simulink model "nms_model_Push"  (R2019a)
settings: Solver=ode15s  StartTime=0.0  StopTime=10  FixedStep=1e-3  MaxStep=ts_max  RelTol=1e-3  AbsTol=1e-4  EnableMultiTasking=on
InitFcn:
  | nms_model_MechInit
  | nms_model_ControlInit
values from neighbouring files (symbols this model uses):
  GainDeltaTheta = 2 /100*180/pi    (= 1.14591559026)    [nms_model_ControlInit.m]
  GainGAS = 1.1/FmaxGAS    [nms_model_ControlInit.m]
  GainGLU = 0.5/FmaxGLU    [nms_model_ControlInit.m]
  GainHAM = 0.65/FmaxHAM    [nms_model_ControlInit.m]
  GainHAMHFL = 4    [nms_model_ControlInit.m]
  GainHFL = 0.5    [nms_model_ControlInit.m]
  GainKneOverExt = 2    [nms_model_ControlInit.m]
  GainSOL = 1.2/FmaxSOL    [nms_model_ControlInit.m]
  GainSOLTA = 0.4/FmaxSOL    [nms_model_ControlInit.m]
  GainTA = 1.1    [nms_model_ControlInit.m]
  GainVAS = 1.2/FmaxVAS    [nms_model_ControlInit.m]
  K_swing = 0.25    [nms_model_ControlInit.m]
  KneePh23Offset = 170*pi/180    (= 2.96705972839)    [nms_model_ControlInit.m]
  LceOffsetHAM = 0.85    [nms_model_ControlInit.m]
  LceOffsetHFL = 0.65    [nms_model_ControlInit.m]
  LceOffsetTA = 1-0.5*w    [nms_model_ControlInit.m]
  LongDelay = 0.020    (= 0.02)    [nms_model_ControlInit.m]
  MidDelay = 0.010    (= 0.01)    [nms_model_ControlInit.m]
  PosGainGG = 1/(30*pi/180)    (= 1.9098593171)    [nms_model_ControlInit.m]
  PreStimGAS = 0.01    [nms_model_ControlInit.m]
  PreStimGG = 0.05    [nms_model_ControlInit.m]
  PreStimGLU = 0.01    [nms_model_ControlInit.m]
  PreStimHAM = 0.01    [nms_model_ControlInit.m]
  PreStimHFL = 0.01    [nms_model_ControlInit.m]
  PreStimSOL = 0.01    [nms_model_ControlInit.m]
  PreStimTA = 0.01    [nms_model_ControlInit.m]
  PreStimVAS = 0.08    [nms_model_ControlInit.m]
  ShortDelay = 0.005    [nms_model_ControlInit.m]
  SpeedGainGG = 0.2    [nms_model_ControlInit.m]
  Theta0 = 6*pi/180    (= 0.10471975512)    [nms_model_ControlInit.m]
undefined symbols (not defined in the file or in its folder): c, c_jointstop, D12_F, D12_S, D12_T, D13_F, D1G_F, D1G_HAT, D1G_S, D1G_T, DeltaThRef, disturbances, dt_visual, eref, FmaxGAS, FmaxGLU, FmaxHAM, FmaxHFL, FmaxSOL, FmaxTA, FmaxVAS, In_F, In_HAT, In_S, In_T, K, k_gx, k_gy, k_pressure, loptGAS, loptGLU, loptHAM, loptHFL, loptSOL, loptTA, loptVAS, lslackGAS, lslackGLU, lslackHAM, lslackHFL, lslackSOL, lslackTA, lslackVAS, m_F, m_HAT, m_S, m_T, mu_slide, mu_stick, N, phi12_LowLimit, phi12_UpLimit, phi23_UpLimit, phi34_UpLimit, phimaxGASa, phimaxGASk, phimaxHAMk, phimaxSOL, phimaxTA, phimaxVAS ... (+44)
libraries: mblibv1 x69, simulink x22, simulink_extras x20, myLibrary2019a x3, myLibrary x1
(part 4 of 8)

== system nms_model_Push/Muscle Actuation Layer/L GAS ==
  note: SOLEUS Muscle-Tendon Dynamics
  note: Excitation Contraction Coupling
  STIM : Inport
  lmtc [m] : Inport  Port=2
  1 : Product  Inputs=**  SaturateOnIntegerOverflow=on  InputSameDT=on  OutDataTypeStr=Inherit: Same as first input
  1/lslack : Gain  Gain=1/lslackGAS  SaturateOnIntegerOverflow=on  OutDataTypeStr=Inherit: Same as input  ParamDataTypeStr=Inherit: Same as input
  BE force-length relation : Subsystem
  CE force-length relation : Subsystem
  CE inverse force-velocity relation : Subsystem
  Constant : Constant  Value=lslackGAS
  ECC TransferFcn : simulink_extras/Additional Linear/Transfer Fcn (with initial outputs)  N=[1]  D="[tau  1]"  Y0=preA  U0=0
      settings: AttributesFormatString=pre-activation: %<Y0>
  Fmax : Gain  Gain=FmaxGAS  SaturateOnIntegerOverflow=on  OutDataTypeStr=Inherit: Same as input  ParamDataTypeStr=Inherit: Same as input
  Fv = Fse / (A*Fce) : Product  Inputs=*/  SaturateOnIntegerOverflow=on  InputSameDT=on  OutDataTypeStr=Inherit: Same as first input
  Integrator : Integrator  InitialConditionSource=external  LowerSaturationLimit=0.05
  PE force-length relation : Subsystem
  SE force-length relation : Subsystem
  Sum : Sum  Inputs=|+-  SaturateOnIntegerOverflow=on  InputSameDT=on  OutDataTypeStr=Inherit: Same as first input
  Sum2 : Sum  Inputs=|-+  SaturateOnIntegerOverflow=on  InputSameDT=on  OutDataTypeStr=Inherit: Same as first input
  Sum3 : Sum  SaturateOnIntegerOverflow=on  InputSameDT=on  OutDataTypeStr=Inherit: Same as first input
  Sum4 : Sum  SaturateOnIntegerOverflow=on  InputSameDT=on  OutDataTypeStr=Inherit: Same as first input
  lce/lopt : Gain  Gain=1/loptGAS  SaturateOnIntegerOverflow=on  OutDataTypeStr=Inherit: Same as input  ParamDataTypeStr=Inherit: Same as input
  vmax*lopt : Gain  Gain=vmaxGAS*loptGAS  SaturateOnIntegerOverflow=on  OutDataTypeStr=Inherit: Same as input  ParamDataTypeStr=Inherit: Same as input
  Fmtc : Outport  InitialOutput=0  VectorParamsAs1DForOutWhenUnconnected=on
  Lce : Outport  Port=2  InitialOutput=0  VectorParamsAs1DForOutWhenUnconnected=on
  Vce : Outport  Port=3  InitialOutput=0  VectorParamsAs1DForOutWhenUnconnected=on
  Lse : Outport  Port=4  InitialOutput=0  VectorParamsAs1DForOutWhenUnconnected=on
  A : Outport  Port=5  InitialOutput=0  VectorParamsAs1DForOutWhenUnconnected=on
  wires:
  Integrator/1 -> Sum/2, lce/lopt/1, Lce/1  "lce"
  Sum/1 -> 1/lslack/1, Lse/1  "lse"
  lce/lopt/1 -> CE force-length relation/1(lce [lopt]), BE force-length relation/1(lce [lopt]), PE force-length relation/1(lce [lopt])
  Fv = Fse / (A*Fce)/1 -> CE inverse force-velocity relation/1(Fv[Fmax])  "fv"
  vmax*lopt/1 -> Integrator/1, Vce/1  "vce"
  lmtc [m]/1 -> Sum2/2, Sum/1  "lmtc"
  Fmax/1 -> Fmtc/1  "Fmtc"
  1/lslack/1 -> SE force-length relation/1(lse [lslack])
  SE force-length relation/1(fse [Fmax]) -> Fmax/1, Sum4/1
  Sum2/1 -> Integrator/2
  Constant/1 -> Sum2/1
  CE force-length relation/1(fce [Fmax]) -> 1/1
  Sum4/1 -> Fv = Fse / (A*Fce)/1
  PE force-length relation/1(fpe [Fmax]) -> Sum3/1
  1/1 -> Sum3/2
  BE force-length relation/1(fbe [Fmax]) -> Sum4/2
  Sum3/1 -> Fv = Fse / (A*Fce)/2
  CE inverse force-velocity relation/1(v[vmax]) -> vmax*lopt/1
  STIM/1 -> ECC TransferFcn/1
  ECC TransferFcn/1 -> A/1, 1/2

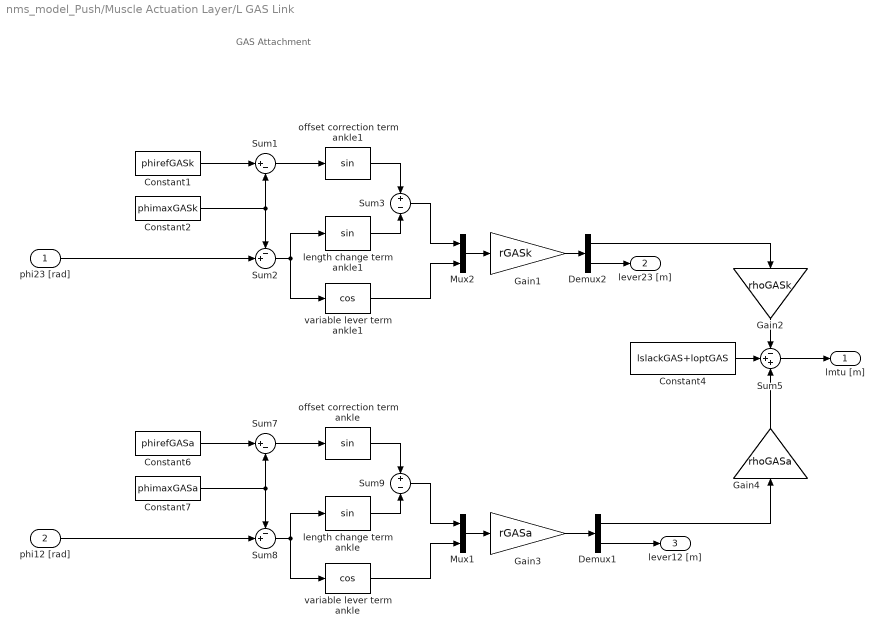
== system nms_model_Push/Muscle Actuation Layer/L GAS Link ==
  note: GAS Attachment
  phi23 [rad] : Inport
  phi12 [rad] : Inport  Port=2
  Constant1 : Constant  Value=phirefGASk
  Constant2 : Constant  Value=phimaxGASk
  Constant4 : Constant  Value=lslackGAS+loptGAS
  Constant6 : Constant  Value=phirefGASa
  Constant7 : Constant  Value=phimaxGASa
  Demux1 : Demux  Outputs=2
  Demux2 : Demux  Outputs=2
  Gain1 : Gain  Gain=rGASk
  Gain2 : Gain  Gain=rhoGASk
  Gain3 : Gain  Gain=rGASa
  Gain4 : Gain  Gain=rhoGASa
  Mux1 : Mux  Inputs=2
  Mux2 : Mux  Inputs=2
  Sum1 : Sum  Inputs=|+-
  Sum2 : Sum  Inputs=-+|
  Sum3 : Sum  Inputs=+-
  Sum5 : Sum  Inputs=-++
  Sum7 : Sum  Inputs=|+-
  Sum8 : Sum  Inputs=-+|
  Sum9 : Sum  Inputs=+-
  length change term ankle : Trigonometry
  length change term ankle1 : Trigonometry
  offset correction term ankle : Trigonometry
  offset correction term ankle1 : Trigonometry
  variable lever term ankle : Trigonometry  Operator=cos
  variable lever term ankle1 : Trigonometry  Operator=cos
  lmtu [m] : Outport  VectorParamsAs1DForOutWhenUnconnected=on
  lever23 [m] : Outport  Port=2  VectorParamsAs1DForOutWhenUnconnected=on
  lever12 [m] : Outport  Port=3  VectorParamsAs1DForOutWhenUnconnected=on
  wires:
  phi12 [rad]/1 -> Sum8/2
  Sum5/1 -> lmtu [m]/1
  variable lever term ankle/1 -> Mux1/2
  Demux1/2 -> lever12 [m]/1
  Sum8/1 -> variable lever term ankle/1, length change term ankle/1
  Constant7/1 -> Sum8/1, Sum7/2
  Sum7/1 -> offset correction term ankle/1
  Constant6/1 -> Sum7/1
  length change term ankle/1 -> Sum9/2
  offset correction term ankle/1 -> Sum9/1
  Sum9/1 -> Mux1/1
  Constant4/1 -> Sum5/2
  Mux1/1 -> Gain3/1
  Gain3/1 -> Demux1/1
  Demux1/1 -> Gain4/1
  Gain4/1 -> Sum5/3
  phi23 [rad]/1 -> Sum2/2
  variable lever term ankle1/1 -> Mux2/2
  Sum2/1 -> variable lever term ankle1/1, length change term ankle1/1
  Constant2/1 -> Sum2/1, Sum1/2
  Sum1/1 -> offset correction term ankle1/1
  Constant1/1 -> Sum1/1
  length change term ankle1/1 -> Sum3/2
  offset correction term ankle1/1 -> Sum3/1
  Sum3/1 -> Mux2/1
  Mux2/1 -> Gain1/1
  Gain1/1 -> Demux2/1
  Demux2/2 -> lever23 [m]/1
  Demux2/1 -> Gain2/1
  Gain2/1 -> Sum5/1

== system nms_model_Push/Muscle Actuation Layer/L GLU ==
  note: SOLEUS Muscle-Tendon Dynamics
  note: Excitation Contraction Coupling
  STIM : Inport
  lmtc [m] : Inport  Port=2
  1 : Product  Inputs=**  SaturateOnIntegerOverflow=on  InputSameDT=on  OutDataTypeStr=Inherit: Same as first input
  1/lslack : Gain  Gain=1/lslackGLU  SaturateOnIntegerOverflow=on  OutDataTypeStr=Inherit: Same as input  ParamDataTypeStr=Inherit: Same as input
  BE force-length relation : Subsystem
  CE force-length relation : Subsystem
  CE inverse force-velocity relation : Subsystem
  Constant : Constant  Value=lslackGLU
  ECC TransferFcn : simulink_extras/Additional Linear/Transfer Fcn (with initial outputs)  N=[1]  D="[tau  1]"  Y0=preA  U0=0
      settings: AttributesFormatString=pre-activation: %<Y0>
  Fmax : Gain  Gain=FmaxGLU  SaturateOnIntegerOverflow=on  OutDataTypeStr=Inherit: Same as input  ParamDataTypeStr=Inherit: Same as input
  Fv = Fse / (A*Fce) : Product  Inputs=*/  SaturateOnIntegerOverflow=on  InputSameDT=on  OutDataTypeStr=Inherit: Same as first input
  Integrator : Integrator  InitialConditionSource=external  LowerSaturationLimit=0.05
  PE force-length relation : Subsystem
  SE force-length relation : Subsystem
  Sum : Sum  Inputs=|+-  SaturateOnIntegerOverflow=on  InputSameDT=on  OutDataTypeStr=Inherit: Same as first input
  Sum2 : Sum  Inputs=|-+  SaturateOnIntegerOverflow=on  InputSameDT=on  OutDataTypeStr=Inherit: Same as first input
  Sum3 : Sum  SaturateOnIntegerOverflow=on  InputSameDT=on  OutDataTypeStr=Inherit: Same as first input
  Sum4 : Sum  SaturateOnIntegerOverflow=on  InputSameDT=on  OutDataTypeStr=Inherit: Same as first input
  lce/lopt : Gain  Gain=1/loptGLU  SaturateOnIntegerOverflow=on  OutDataTypeStr=Inherit: Same as input  ParamDataTypeStr=Inherit: Same as input
  vmax*lopt : Gain  Gain=vmaxGLU*loptGLU  SaturateOnIntegerOverflow=on  OutDataTypeStr=Inherit: Same as input  ParamDataTypeStr=Inherit: Same as input
  Fmtc : Outport  InitialOutput=0  VectorParamsAs1DForOutWhenUnconnected=on
  Lce : Outport  Port=2  InitialOutput=0  VectorParamsAs1DForOutWhenUnconnected=on
  Vce : Outport  Port=3  InitialOutput=0  VectorParamsAs1DForOutWhenUnconnected=on
  Lse : Outport  Port=4  InitialOutput=0  VectorParamsAs1DForOutWhenUnconnected=on
  A : Outport  Port=5  InitialOutput=0  VectorParamsAs1DForOutWhenUnconnected=on
  wires:
  Integrator/1 -> Sum/2, lce/lopt/1, Lce/1  "lce"
  Sum/1 -> 1/lslack/1, Lse/1  "lse"
  lce/lopt/1 -> CE force-length relation/1(lce [lopt]), BE force-length relation/1(lce [lopt]), PE force-length relation/1(lce [lopt])
  Fv = Fse / (A*Fce)/1 -> CE inverse force-velocity relation/1(Fv[Fmax])  "fv"
  vmax*lopt/1 -> Integrator/1, Vce/1  "vce"
  lmtc [m]/1 -> Sum2/2, Sum/1  "lmtc"
  Fmax/1 -> Fmtc/1  "Fmtc"
  1/lslack/1 -> SE force-length relation/1(lse [lslack])
  SE force-length relation/1(fse [Fmax]) -> Fmax/1, Sum4/1
  Sum2/1 -> Integrator/2
  Constant/1 -> Sum2/1
  CE force-length relation/1(fce [Fmax]) -> 1/1
  Sum4/1 -> Fv = Fse / (A*Fce)/1
  PE force-length relation/1(fpe [Fmax]) -> Sum3/1
  1/1 -> Sum3/2
  BE force-length relation/1(fbe [Fmax]) -> Sum4/2
  Sum3/1 -> Fv = Fse / (A*Fce)/2
  CE inverse force-velocity relation/1(v[vmax]) -> vmax*lopt/1
  STIM/1 -> ECC TransferFcn/1
  ECC TransferFcn/1 -> A/1, 1/2

== system nms_model_Push/Muscle Actuation Layer/L GLU Link ==
  note: GLUTEUS Attachment
  phi34 [rad] : Inport
  Constant : Constant  Value=lslackGLU+loptGLU
  Constant1 : Constant  Value=rGLU
  Constant2 : Constant  Value=phirefGLU
  Gain2 : Gain  Gain=rhoGLU
  Product : Product  RndMeth=Zero
  Sum2 : Sum  Inputs=|+-
  Sum5 : Sum  Inputs=|+-
  lmtu [m] : Outport  VectorParamsAs1DForOutWhenUnconnected=on
  lever [m] : Outport  Port=2  VectorParamsAs1DForOutWhenUnconnected=on
  wires:
  Constant/1 -> Sum5/1
  Sum5/1 -> lmtu [m]/1
  Product/1 -> Gain2/1
  phi34 [rad]/1 -> Sum2/1
  Constant2/1 -> Sum2/2
  Sum2/1 -> Product/1
  Constant1/1 -> Product/2, lever [m]/1
  Gain2/1 -> Sum5/2

== system nms_model_Push/Muscle Actuation Layer/L HAM ==
  note: SOLEUS Muscle-Tendon Dynamics
  note: Excitation Contraction Coupling
  STIM : Inport
  lmtc [m] : Inport  Port=2
  1 : Product  Inputs=**  SaturateOnIntegerOverflow=on  InputSameDT=on  OutDataTypeStr=Inherit: Same as first input
  1/lslack : Gain  Gain=1/lslackHAM  SaturateOnIntegerOverflow=on  OutDataTypeStr=Inherit: Same as input  ParamDataTypeStr=Inherit: Same as input
  BE force-length relation : Subsystem
  CE force-length relation : Subsystem
  CE inverse force-velocity relation : Subsystem
  Constant : Constant  Value=lslackHAM
  ECC TransferFcn : simulink_extras/Additional Linear/Transfer Fcn (with initial outputs)  N=[1]  D="[tau  1]"  Y0=preA  U0=0
      settings: AttributesFormatString=pre-activation: %<Y0>
  Fmax : Gain  Gain=FmaxHAM  SaturateOnIntegerOverflow=on  OutDataTypeStr=Inherit: Same as input  ParamDataTypeStr=Inherit: Same as input
  Fv = Fse / (A*Fce) : Product  Inputs=*/  SaturateOnIntegerOverflow=on  InputSameDT=on  OutDataTypeStr=Inherit: Same as first input
  Integrator : Integrator  InitialConditionSource=external  LowerSaturationLimit=0.05
  PE force-length relation : Subsystem
  SE force-length relation : Subsystem
  Sum : Sum  Inputs=|+-  SaturateOnIntegerOverflow=on  InputSameDT=on  OutDataTypeStr=Inherit: Same as first input
  Sum2 : Sum  Inputs=|-+  SaturateOnIntegerOverflow=on  InputSameDT=on  OutDataTypeStr=Inherit: Same as first input
  Sum3 : Sum  SaturateOnIntegerOverflow=on  InputSameDT=on  OutDataTypeStr=Inherit: Same as first input
  Sum4 : Sum  SaturateOnIntegerOverflow=on  InputSameDT=on  OutDataTypeStr=Inherit: Same as first input
  lce/lopt : Gain  Gain=1/loptHAM  SaturateOnIntegerOverflow=on  OutDataTypeStr=Inherit: Same as input  ParamDataTypeStr=Inherit: Same as input
  vmax*lopt : Gain  Gain=vmaxHAM*loptHAM  SaturateOnIntegerOverflow=on  OutDataTypeStr=Inherit: Same as input  ParamDataTypeStr=Inherit: Same as input
  Fmtc : Outport  InitialOutput=0  VectorParamsAs1DForOutWhenUnconnected=on
  Lce : Outport  Port=2  InitialOutput=0  VectorParamsAs1DForOutWhenUnconnected=on
  Vce : Outport  Port=3  InitialOutput=0  VectorParamsAs1DForOutWhenUnconnected=on
  Lse : Outport  Port=4  InitialOutput=0  VectorParamsAs1DForOutWhenUnconnected=on
  A : Outport  Port=5  InitialOutput=0  VectorParamsAs1DForOutWhenUnconnected=on
  wires:
  Integrator/1 -> Sum/2, lce/lopt/1, Lce/1  "lce"
  Sum/1 -> 1/lslack/1, Lse/1  "lse"
  lce/lopt/1 -> CE force-length relation/1(lce [lopt]), BE force-length relation/1(lce [lopt]), PE force-length relation/1(lce [lopt])
  Fv = Fse / (A*Fce)/1 -> CE inverse force-velocity relation/1(Fv[Fmax])  "fv"
  vmax*lopt/1 -> Integrator/1, Vce/1  "vce"
  lmtc [m]/1 -> Sum2/2, Sum/1  "lmtc"
  Fmax/1 -> Fmtc/1  "Fmtc"
  1/lslack/1 -> SE force-length relation/1(lse [lslack])
  SE force-length relation/1(fse [Fmax]) -> Fmax/1, Sum4/1
  Sum2/1 -> Integrator/2
  Constant/1 -> Sum2/1
  CE force-length relation/1(fce [Fmax]) -> 1/1
  Sum4/1 -> Fv = Fse / (A*Fce)/1
  PE force-length relation/1(fpe [Fmax]) -> Sum3/1
  1/1 -> Sum3/2
  BE force-length relation/1(fbe [Fmax]) -> Sum4/2
  Sum3/1 -> Fv = Fse / (A*Fce)/2
  CE inverse force-velocity relation/1(v[vmax]) -> vmax*lopt/1
  STIM/1 -> ECC TransferFcn/1
  ECC TransferFcn/1 -> 1/2, A/1

== system nms_model_Push/Muscle Actuation Layer/L HAM Link ==
  note: HAM Attachment
  phi34 [rad] : Inport
  phi23 [rad] : Inport  Port=2
  Constant3 : Constant  Value=rHAMh
  Constant4 : Constant  Value=lslackHAM+loptHAM
  Constant5 : Constant  Value=phirefHAMh
  Constant6 : Constant  Value=phirefHAMk
  Constant7 : Constant  Value=phimaxHAMk  VectorParams1D=off
  Demux1 : Demux  Outputs=2
  Gain2 : Gain  Gain=rhoHAMh
  Gain3 : Gain  Gain=rHAMk
  Gain4 : Gain  Gain=rhoHAMk
  Mux1 : Mux  Inputs=2
  Product : Product  RndMeth=Zero
  Sum4 : Sum  Inputs=|+-
  Sum5 : Sum  Inputs=-+-
  Sum7 : Sum  Inputs=|+-
  Sum8 : Sum  Inputs=-+|
  Sum9 : Sum  Inputs=+-
  length change term ankle : Trigonometry
  offset correction term ankle : Trigonometry
  variable lever term ankle : Trigonometry  Operator=cos
  lmtu [m] : Outport  VectorParamsAs1DForOutWhenUnconnected=on
  lever34 [m] : Outport  Port=2  VectorParamsAs1DForOutWhenUnconnected=on
  lever23 [m] : Outport  Port=3  VectorParamsAs1DForOutWhenUnconnected=on
  wires:
  phi23 [rad]/1 -> Sum8/2
  Sum5/1 -> lmtu [m]/1
  variable lever term ankle/1 -> Mux1/2
  Demux1/2 -> lever23 [m]/1
  Sum8/1 -> variable lever term ankle/1, length change term ankle/1
  Constant7/1 -> Sum8/1, Sum7/2
  Sum7/1 -> offset correction term ankle/1
  Constant6/1 -> Sum7/1
  length change term ankle/1 -> Sum9/2
  offset correction term ankle/1 -> Sum9/1
  Sum9/1 -> Mux1/1
  Constant4/1 -> Sum5/2
  Mux1/1 -> Gain3/1
  Gain3/1 -> Demux1/1
  Demux1/1 -> Gain4/1
  Gain4/1 -> Sum5/3
  Gain2/1 -> Sum5/1
  phi34 [rad]/1 -> Sum4/1
  Constant5/1 -> Sum4/2
  Sum4/1 -> Product/1
  Constant3/1 -> Product/2, lever34 [m]/1
  Product/1 -> Gain2/1

== system nms_model_Push/Muscle Actuation Layer/L HFL ==
  note: SOLEUS Muscle-Tendon Dynamics
  note: Excitation Contraction Coupling
  STIM : Inport
  lmtc [m] : Inport  Port=2
  1 : Product  Inputs=**  SaturateOnIntegerOverflow=on  InputSameDT=on  OutDataTypeStr=Inherit: Same as first input
  1/lslack : Gain  Gain=1/lslackHFL  SaturateOnIntegerOverflow=on  OutDataTypeStr=Inherit: Same as input  ParamDataTypeStr=Inherit: Same as input
  BE force-length relation : Subsystem
  CE force-length relation : Subsystem
  CE inverse force-velocity relation : Subsystem
  Constant : Constant  Value=lslackHFL
  ECC TransferFcn : simulink_extras/Additional Linear/Transfer Fcn (with initial outputs)  N=[1]  D="[tau  1]"  Y0=preA  U0=0
      settings: AttributesFormatString=pre-activation: %<Y0>
  Fmax : Gain  Gain=FmaxHFL  SaturateOnIntegerOverflow=on  OutDataTypeStr=Inherit: Same as input  ParamDataTypeStr=Inherit: Same as input
  Fv = Fse / (A*Fce) : Product  Inputs=*/  SaturateOnIntegerOverflow=on  InputSameDT=on  OutDataTypeStr=Inherit: Same as first input
  Integrator : Integrator  InitialConditionSource=external  LowerSaturationLimit=0.05
  PE force-length relation : Subsystem
  SE force-length relation : Subsystem
  Sum : Sum  Inputs=|+-  SaturateOnIntegerOverflow=on  InputSameDT=on  OutDataTypeStr=Inherit: Same as first input
  Sum2 : Sum  Inputs=|-+  SaturateOnIntegerOverflow=on  InputSameDT=on  OutDataTypeStr=Inherit: Same as first input
  Sum3 : Sum  SaturateOnIntegerOverflow=on  InputSameDT=on  OutDataTypeStr=Inherit: Same as first input
  Sum4 : Sum  SaturateOnIntegerOverflow=on  InputSameDT=on  OutDataTypeStr=Inherit: Same as first input
  lce/lopt : Gain  Gain=1/loptHFL  SaturateOnIntegerOverflow=on  OutDataTypeStr=Inherit: Same as input  ParamDataTypeStr=Inherit: Same as input
  vmax*lopt : Gain  Gain=vmaxHFL*loptHFL  SaturateOnIntegerOverflow=on  OutDataTypeStr=Inherit: Same as input  ParamDataTypeStr=Inherit: Same as input
  Fmtc : Outport  InitialOutput=0  VectorParamsAs1DForOutWhenUnconnected=on
  Lce : Outport  Port=2  InitialOutput=0  VectorParamsAs1DForOutWhenUnconnected=on
  Vce : Outport  Port=3  InitialOutput=0  VectorParamsAs1DForOutWhenUnconnected=on
  Lse : Outport  Port=4  InitialOutput=0  VectorParamsAs1DForOutWhenUnconnected=on
  A : Outport  Port=5  InitialOutput=0  VectorParamsAs1DForOutWhenUnconnected=on
  wires:
  Integrator/1 -> Sum/2, lce/lopt/1, Lce/1  "lce"
  Sum/1 -> 1/lslack/1, Lse/1  "lse"
  lce/lopt/1 -> CE force-length relation/1(lce [lopt]), BE force-length relation/1(lce [lopt]), PE force-length relation/1(lce [lopt])
  Fv = Fse / (A*Fce)/1 -> CE inverse force-velocity relation/1(Fv[Fmax])  "fv"
  vmax*lopt/1 -> Integrator/1, Vce/1  "vce"
  lmtc [m]/1 -> Sum2/2, Sum/1  "lmtc"
  Fmax/1 -> Fmtc/1  "Fmtc"
  1/lslack/1 -> SE force-length relation/1(lse [lslack])
  SE force-length relation/1(fse [Fmax]) -> Fmax/1, Sum4/1
  Sum2/1 -> Integrator/2
  Constant/1 -> Sum2/1
  CE force-length relation/1(fce [Fmax]) -> 1/1
  Sum4/1 -> Fv = Fse / (A*Fce)/1
  PE force-length relation/1(fpe [Fmax]) -> Sum3/1
  1/1 -> Sum3/2
  BE force-length relation/1(fbe [Fmax]) -> Sum4/2
  Sum3/1 -> Fv = Fse / (A*Fce)/2
  CE inverse force-velocity relation/1(v[vmax]) -> vmax*lopt/1
  STIM/1 -> ECC TransferFcn/1
  ECC TransferFcn/1 -> A/1, 1/2

== system nms_model_Push/Muscle Actuation Layer/L HFL Link ==
  note: HFL Attachment
  phi34 [rad] : Inport
  Constant : Constant  Value=lslackHFL+loptHFL
  Constant1 : Constant  Value=rHFL
  Constant2 : Constant  Value=phirefHFL
  Gain2 : Gain  Gain=rhoHFL
  Product : Product  RndMeth=Zero
  Sum2 : Sum  Inputs=|+-
  Sum5 : Sum  Inputs=|++
  lmtu [m] : Outport  VectorParamsAs1DForOutWhenUnconnected=on
  lever [m] : Outport  Port=2  VectorParamsAs1DForOutWhenUnconnected=on
  wires:
  Constant/1 -> Sum5/1
  Sum5/1 -> lmtu [m]/1
  Product/1 -> Gain2/1
  phi34 [rad]/1 -> Sum2/1
  Constant2/1 -> Sum2/2
  Sum2/1 -> Product/1
  Constant1/1 -> Product/2, lever [m]/1
  Gain2/1 -> Sum5/2

== system nms_model_Push/Muscle Actuation Layer/L Hip Joint Limits ==
  note: Ankle Joint Limits
  phi [rad] : Inport
  dphi [rad/s] : Inport  Port=2
  Gain2 : Gain  Gain=-1
  Gain3 : Gain  Gain=c_jointstop
  Gain4 : Gain  Gain=1/w_max_jointstop
  Limit Ankle Range : simulink/Logic and Bit Operations/Interval Test  IntervalClosedRight=on  uplimit=phi34_UpLimit + 30*pi/180  IntervalClosedLeft=on  lowlimit=10*pi/180  OutDataTypeStr=boolean
  Logical Operator3 : Logic  Operator=NOT  AllPortsSameDT=off  OutDataTypeStr=boolean
  Mux3 : Mux  Inputs=2
  Overextension Torque : Fcn  Expr="- u(1)  *  (1-u(2)) * (u(2)<1) * (u(1)>0)"
  Stop Simulation1 : Stop
  Sum : Sum  Inputs=|+-
  overextension angle : Constant  Value=phi34_UpLimit
  M_stop [Nm] : Outport  VectorParamsAs1DForOutWhenUnconnected=on
  wires:
  Mux3/1 -> Overextension Torque/1
  Gain3/1 -> Mux3/1
  dphi [rad/s]/1 -> Gain4/1
  overextension angle/1 -> Sum/2
  phi [rad]/1 -> Sum/1, Limit Ankle Range/1
  Sum/1 -> Gain3/1
  Gain4/1 -> Gain2/1
  Gain2/1 -> Mux3/2
  Overextension Torque/1 -> M_stop [Nm]/1
  Limit Ankle Range/1 -> Logical Operator3/1
  Logical Operator3/1 -> Stop Simulation1/1

== system nms_model_Push/Muscle Actuation Layer/L Knee Joint Limits ==
  note: Ankle Joint Limits
  phi [rad] : Inport
  dphi [rad/s] : Inport  Port=2
  Gain2 : Gain  Gain=-1
  Gain3 : Gain  Gain=c_jointstop
  Gain4 : Gain  Gain=1/w_max_jointstop
  Limit Ankle Range : simulink/Logic and Bit Operations/Interval Test  IntervalClosedRight=on  uplimit=185*pi/180  IntervalClosedLeft=on  lowlimit=40*pi/180  OutDataTypeStr=boolean
  Logical Operator3 : Logic  Operator=NOT  AllPortsSameDT=off  OutDataTypeStr=boolean
  Mux3 : Mux  Inputs=2
  Overextension Torque : Fcn  Expr="- u(1)  *  (1-u(2)) * (u(2)<1) * (u(1)>0)"
  Stop Simulation1 : Stop
  Sum : Sum  Inputs=|+-
  overextension angle : Constant  Value=phi23_UpLimit
  M_stop [Nm] : Outport  VectorParamsAs1DForOutWhenUnconnected=on
  wires:
  Mux3/1 -> Overextension Torque/1
  Gain3/1 -> Mux3/1
  dphi [rad/s]/1 -> Gain4/1
  overextension angle/1 -> Sum/2
  phi [rad]/1 -> Sum/1, Limit Ankle Range/1
  Sum/1 -> Gain3/1
  Gain4/1 -> Gain2/1
  Gain2/1 -> Mux3/2
  Overextension Torque/1 -> M_stop [Nm]/1
  Limit Ankle Range/1 -> Logical Operator3/1
  Logical Operator3/1 -> Stop Simulation1/1

== system nms_model_Push/Muscle Actuation Layer/L SOL ==
  note: SOLEUS Muscle-Tendon Dynamics
  note: Excitation Contraction Coupling
  STIM : Inport
  lmtc [m] : Inport  Port=2
  1 : Product  Inputs=**  SaturateOnIntegerOverflow=on  InputSameDT=on  OutDataTypeStr=Inherit: Same as first input
  1/lslack : Gain  Gain=1/lslackSOL  SaturateOnIntegerOverflow=on  OutDataTypeStr=Inherit: Same as input  ParamDataTypeStr=Inherit: Same as input
  BE force-length relation : Subsystem
  CE force-length relation : Subsystem
  CE inverse force-velocity relation : Subsystem
  Constant : Constant  Value=lslackSOL
  ECC TransferFcn : simulink_extras/Additional Linear/Transfer Fcn (with initial outputs)  N=[1]  D="[tau  1]"  Y0=preA  U0=0
      settings: AttributesFormatString=pre-activation: %<Y0>
  Fmax : Gain  Gain=FmaxSOL  SaturateOnIntegerOverflow=on  OutDataTypeStr=Inherit: Same as input  ParamDataTypeStr=Inherit: Same as input
  Fv = Fse / (A*Fce) : Product  Inputs=*/  SaturateOnIntegerOverflow=on  InputSameDT=on  OutDataTypeStr=Inherit: Same as first input
  Integrator : Integrator  InitialConditionSource=external  LowerSaturationLimit=0.05
  PE force-length relation : Subsystem
  SE force-length relation : Subsystem
  Sum : Sum  Inputs=|+-  SaturateOnIntegerOverflow=on  InputSameDT=on  OutDataTypeStr=Inherit: Same as first input
  Sum2 : Sum  Inputs=|-+  SaturateOnIntegerOverflow=on  InputSameDT=on  OutDataTypeStr=Inherit: Same as first input
  Sum3 : Sum  SaturateOnIntegerOverflow=on  InputSameDT=on  OutDataTypeStr=Inherit: Same as first input
  Sum4 : Sum  SaturateOnIntegerOverflow=on  InputSameDT=on  OutDataTypeStr=Inherit: Same as first input
  lce/lopt : Gain  Gain=1/loptSOL  SaturateOnIntegerOverflow=on  OutDataTypeStr=Inherit: Same as input  ParamDataTypeStr=Inherit: Same as input
  vmax*lopt : Gain  Gain=vmaxSOL*loptSOL  SaturateOnIntegerOverflow=on  OutDataTypeStr=Inherit: Same as input  ParamDataTypeStr=Inherit: Same as input
  Fmtc : Outport  InitialOutput=0  VectorParamsAs1DForOutWhenUnconnected=on
  Lce : Outport  Port=2  InitialOutput=0  VectorParamsAs1DForOutWhenUnconnected=on
  Vce : Outport  Port=3  InitialOutput=0  VectorParamsAs1DForOutWhenUnconnected=on
  Lse : Outport  Port=4  InitialOutput=0  VectorParamsAs1DForOutWhenUnconnected=on
  A : Outport  Port=5  InitialOutput=0  VectorParamsAs1DForOutWhenUnconnected=on
  wires:
  Integrator/1 -> Sum/2, lce/lopt/1, Lce/1  "lce"
  Sum/1 -> 1/lslack/1, Lse/1  "lse"
  lce/lopt/1 -> CE force-length relation/1(lce [lopt]), BE force-length relation/1(lce [lopt]), PE force-length relation/1(lce [lopt])
  Fv = Fse / (A*Fce)/1 -> CE inverse force-velocity relation/1(Fv[Fmax])  "fv"
  vmax*lopt/1 -> Integrator/1, Vce/1  "vce"
  lmtc [m]/1 -> Sum2/2, Sum/1  "lmtc"
  Fmax/1 -> Fmtc/1  "Fmtc"
  1/lslack/1 -> SE force-length relation/1(lse [lslack])
  SE force-length relation/1(fse [Fmax]) -> Fmax/1, Sum4/1
  Sum2/1 -> Integrator/2
  Constant/1 -> Sum2/1
  CE force-length relation/1(fce [Fmax]) -> 1/1
  Sum4/1 -> Fv = Fse / (A*Fce)/1
  PE force-length relation/1(fpe [Fmax]) -> Sum3/1
  1/1 -> Sum3/2
  BE force-length relation/1(fbe [Fmax]) -> Sum4/2
  Sum3/1 -> Fv = Fse / (A*Fce)/2
  CE inverse force-velocity relation/1(v[vmax]) -> vmax*lopt/1
  STIM/1 -> ECC TransferFcn/1
  ECC TransferFcn/1 -> A/1, 1/2

== system nms_model_Push/Muscle Actuation Layer/L SOL Link ==
  note: Soleus Attachment
  phi12 [rad] : Inport
  Constant : Constant  Value=lslackSOL+loptSOL
  Constant2 : Constant  Value=phirefSOL
  Constant3 : Constant  Value=phimaxSOL
  Demux : Demux  Outputs=2
  Gain2 : Gain  Gain=rSOL
  Gain4 : Gain  Gain=rhoSOL
  Mux : Mux  Inputs=2
  Sum2 : Sum  Inputs=|+-
  Sum3 : Sum  Inputs=-+|
  Sum4 : Sum  Inputs=+-
  Sum5 : Sum  Inputs=|++
  length change term : Trigonometry
  offset correction term : Trigonometry
  variable lever term : Trigonometry  Operator=cos
  lmtc [m] : Outport  VectorParamsAs1DForOutWhenUnconnected=on
  lever [m] : Outport  Port=2  VectorParamsAs1DForOutWhenUnconnected=on
  wires:
  phi12 [rad]/1 -> Sum3/2
  Sum3/1 -> variable lever term/1, length change term/1
  Constant3/1 -> Sum3/1, Sum2/2
  Sum2/1 -> offset correction term/1
  Constant2/1 -> Sum2/1
  length change term/1 -> Sum4/2
  offset correction term/1 -> Sum4/1
  Sum4/1 -> Mux/1
  Constant/1 -> Sum5/1
  Sum5/1 -> lmtc [m]/1
  Gain4/1 -> Sum5/2
  variable lever term/1 -> Mux/2
  Mux/1 -> Gain2/1
  Gain2/1 -> Demux/1
  Demux/1 -> Gain4/1
  Demux/2 -> lever [m]/1

== system nms_model_Push/Muscle Actuation Layer/L TA ==
  note: Excitation Contraction Coupling
  note: SOLEUS Muscle-Tendon Dynamics
  STIM : Inport
  lmtc [m] : Inport  Port=2
  1 : Product  Inputs=**  SaturateOnIntegerOverflow=on  InputSameDT=on  OutDataTypeStr=Inherit: Same as first input
  1/lslack : Gain  Gain=1/lslackTA  SaturateOnIntegerOverflow=on  OutDataTypeStr=Inherit: Same as input  ParamDataTypeStr=Inherit: Same as input
  BE force-length relation : Subsystem
  CE force-length relation : Subsystem
  CE inverse force-velocity relation : Subsystem
  Constant : Constant  Value=lslackTA
  ECC TransferFcn : simulink_extras/Additional Linear/Transfer Fcn (with initial outputs)  N=[1]  D="[tau  1]"  Y0=preA  U0=0
      settings: AttributesFormatString=pre-activation: %<Y0>
  Fmax : Gain  Gain=FmaxTA  SaturateOnIntegerOverflow=on  OutDataTypeStr=Inherit: Same as input  ParamDataTypeStr=Inherit: Same as input
  Fv = Fse / (A*Fce) : Product  Inputs=*/  SaturateOnIntegerOverflow=on  InputSameDT=on  OutDataTypeStr=Inherit: Same as first input
  Integrator : Integrator  InitialConditionSource=external  LowerSaturationLimit=0.05
  PE force-length relation : Subsystem
  SE force-length relation : Subsystem
  Sum : Sum  Inputs=|+-  SaturateOnIntegerOverflow=on  InputSameDT=on  OutDataTypeStr=Inherit: Same as first input
  Sum2 : Sum  Inputs=|-+  SaturateOnIntegerOverflow=on  InputSameDT=on  OutDataTypeStr=Inherit: Same as first input
  Sum3 : Sum  SaturateOnIntegerOverflow=on  InputSameDT=on  OutDataTypeStr=Inherit: Same as first input
  Sum4 : Sum  SaturateOnIntegerOverflow=on  InputSameDT=on  OutDataTypeStr=Inherit: Same as first input
  lce/lopt : Gain  Gain=1/loptTA  SaturateOnIntegerOverflow=on  OutDataTypeStr=Inherit: Same as input  ParamDataTypeStr=Inherit: Same as input
  vmax*lopt : Gain  Gain=vmaxTA*loptTA  SaturateOnIntegerOverflow=on  OutDataTypeStr=Inherit: Same as input  ParamDataTypeStr=Inherit: Same as input
  Fmtc : Outport  InitialOutput=0  VectorParamsAs1DForOutWhenUnconnected=on
  Lce : Outport  Port=2  InitialOutput=0  VectorParamsAs1DForOutWhenUnconnected=on
  Vce : Outport  Port=3  InitialOutput=0  VectorParamsAs1DForOutWhenUnconnected=on
  Lse : Outport  Port=4  InitialOutput=0  VectorParamsAs1DForOutWhenUnconnected=on
  A : Outport  Port=5  InitialOutput=0  VectorParamsAs1DForOutWhenUnconnected=on
  wires:
  CE inverse force-velocity relation/1(v[vmax]) -> vmax*lopt/1
  Sum3/1 -> Fv = Fse / (A*Fce)/2
  BE force-length relation/1(fbe [Fmax]) -> Sum4/2
  1/1 -> Sum3/2
  PE force-length relation/1(fpe [Fmax]) -> Sum3/1
  Sum4/1 -> Fv = Fse / (A*Fce)/1
  CE force-length relation/1(fce [Fmax]) -> 1/1
  Constant/1 -> Sum2/1
  Sum2/1 -> Integrator/2
  SE force-length relation/1(fse [Fmax]) -> Sum4/1, Fmax/1
  1/lslack/1 -> SE force-length relation/1(lse [lslack])
  Fmax/1 -> Fmtc/1  "Fmtc"
  lmtc [m]/1 -> Sum/1, Sum2/2  "lmtc"
  vmax*lopt/1 -> Integrator/1, Vce/1  "vce"
  Fv = Fse / (A*Fce)/1 -> CE inverse force-velocity relation/1(Fv[Fmax])  "fv"
  lce/lopt/1 -> BE force-length relation/1(lce [lopt]), PE force-length relation/1(lce [lopt]), CE force-length relation/1(lce [lopt])
  Sum/1 -> Lse/1, 1/lslack/1  "lse"
  Integrator/1 -> lce/lopt/1, Sum/2, Lce/1  "lce"
  STIM/1 -> ECC TransferFcn/1
  ECC TransferFcn/1 -> 1/2, A/1

== system nms_model_Push/Muscle Actuation Layer/L TA Link ==
  note: Muscle Length and Moment Arm
  phi12 [rad] : Inport
  Constant : Constant  Value=lslackTA+loptTA
  Constant2 : Constant  Value=phirefTA
  Constant3 : Constant  Value=phimaxTA
  Demux : Demux  Outputs=2
  Gain2 : Gain  Gain=rTA
  Gain4 : Gain  Gain=rhoTA
  Mux : Mux  Inputs=2
  Sum2 : Sum  Inputs=|+-
  Sum3 : Sum  Inputs=-+|
  Sum4 : Sum  Inputs=+-
  Sum5 : Sum  Inputs=|+-
  length change term : Trigonometry
  offset correction term : Trigonometry
  variable lever term : Trigonometry  Operator=cos
  lmtc [m] : Outport  VectorParamsAs1DForOutWhenUnconnected=on
  lever [m] : Outport  Port=2  VectorParamsAs1DForOutWhenUnconnected=on
  wires:
  phi12 [rad]/1 -> Sum3/2
  Sum3/1 -> variable lever term/1, length change term/1
  Constant3/1 -> Sum3/1, Sum2/2
  Sum2/1 -> offset correction term/1
  Constant2/1 -> Sum2/1
  length change term/1 -> Sum4/2
  offset correction term/1 -> Sum4/1
  Sum4/1 -> Mux/1
  Constant/1 -> Sum5/1
  Sum5/1 -> lmtc [m]/1
  Gain4/1 -> Sum5/2
  variable lever term/1 -> Mux/2
  Mux/1 -> Gain2/1
  Gain2/1 -> Demux/1
  Demux/1 -> Gain4/1
  Demux/2 -> lever [m]/1

== system nms_model_Push/Muscle Actuation Layer/L VAS ==
  note: VASTI Muscle-Tendon Dynamics
  note: Excitation Contraction Coupling
  STIM : Inport
  lmtc [m] : Inport  Port=2
  1 : Product  Inputs=**  SaturateOnIntegerOverflow=on  InputSameDT=on  OutDataTypeStr=Inherit: Same as first input
  1/lslack : Gain  Gain=1/lslackVAS  SaturateOnIntegerOverflow=on  OutDataTypeStr=Inherit: Same as input  ParamDataTypeStr=Inherit: Same as input
  BE force-length relation : Subsystem
  CE force-length relation : Subsystem
  CE inverse force-velocity relation : Subsystem
  Constant : Constant  Value=lslackVAS
  ECC TransferFcn : simulink_extras/Additional Linear/Transfer Fcn (with initial outputs)  N=[1]  D="[tau  1]"  Y0=preA  U0=0
      settings: AttributesFormatString=pre-activation: %<Y0>
  Fmax : Gain  Gain=FmaxVAS  SaturateOnIntegerOverflow=on  OutDataTypeStr=Inherit: Same as input  ParamDataTypeStr=Inherit: Same as input
  Fv = Fse / (A*Fce) : Product  Inputs=*/  SaturateOnIntegerOverflow=on  InputSameDT=on  OutDataTypeStr=Inherit: Same as first input
  Integrator : Integrator  InitialConditionSource=external  LowerSaturationLimit=0.05
  PE force-length relation : Subsystem
  SE force-length relation : Subsystem
  Sum : Sum  Inputs=|+-  SaturateOnIntegerOverflow=on  InputSameDT=on  OutDataTypeStr=Inherit: Same as first input
  Sum2 : Sum  Inputs=|-+  SaturateOnIntegerOverflow=on  InputSameDT=on  OutDataTypeStr=Inherit: Same as first input
  Sum3 : Sum  SaturateOnIntegerOverflow=on  InputSameDT=on  OutDataTypeStr=Inherit: Same as first input
  Sum4 : Sum  SaturateOnIntegerOverflow=on  InputSameDT=on  OutDataTypeStr=Inherit: Same as first input
  lce/lopt : Gain  Gain=1/loptVAS  SaturateOnIntegerOverflow=on  OutDataTypeStr=Inherit: Same as input  ParamDataTypeStr=Inherit: Same as input
  vmax*lopt : Gain  Gain=vmaxVAS*loptVAS  SaturateOnIntegerOverflow=on  OutDataTypeStr=Inherit: Same as input  ParamDataTypeStr=Inherit: Same as input
  Fmtc : Outport  InitialOutput=0  VectorParamsAs1DForOutWhenUnconnected=on
  Lce : Outport  Port=2  InitialOutput=0  VectorParamsAs1DForOutWhenUnconnected=on
  Vce : Outport  Port=3  InitialOutput=0  VectorParamsAs1DForOutWhenUnconnected=on
  Lse : Outport  Port=4  InitialOutput=0  VectorParamsAs1DForOutWhenUnconnected=on
  A : Outport  Port=5  InitialOutput=0  VectorParamsAs1DForOutWhenUnconnected=on
  wires:
  Integrator/1 -> Sum/2, lce/lopt/1, Lce/1  "lce"
  Sum/1 -> 1/lslack/1, Lse/1  "lse"
  lce/lopt/1 -> CE force-length relation/1(lce [lopt]), BE force-length relation/1(lce [lopt]), PE force-length relation/1(lce [lopt])
  Fv = Fse / (A*Fce)/1 -> CE inverse force-velocity relation/1(Fv[Fmax])  "fv"
  vmax*lopt/1 -> Integrator/1, Vce/1  "vce"
  lmtc [m]/1 -> Sum2/2, Sum/1  "lmtc"
  Fmax/1 -> Fmtc/1  "Fmtc"
  1/lslack/1 -> SE force-length relation/1(lse [lslack])
  SE force-length relation/1(fse [Fmax]) -> Fmax/1, Sum4/1
  Sum2/1 -> Integrator/2
  Constant/1 -> Sum2/1
  CE force-length relation/1(fce [Fmax]) -> 1/1
  Sum4/1 -> Fv = Fse / (A*Fce)/1
  PE force-length relation/1(fpe [Fmax]) -> Sum3/1
  1/1 -> Sum3/2
  BE force-length relation/1(fbe [Fmax]) -> Sum4/2
  Sum3/1 -> Fv = Fse / (A*Fce)/2
  CE inverse force-velocity relation/1(v[vmax]) -> vmax*lopt/1
  STIM/1 -> ECC TransferFcn/1
  ECC TransferFcn/1 -> 1/2, A/1

== system nms_model_Push/Muscle Actuation Layer/L VAS Link ==
  note: Muscle Length and Moment Arm
  phi23 [rad] : Inport
  Constant : Constant  Value=lslackVAS+loptVAS
  Constant2 : Constant  Value=phirefVAS
  Constant3 : Constant  Value=phimaxVAS
  Demux : Demux  Outputs=2
  Gain2 : Gain  Gain=rVAS
  Gain4 : Gain  Gain=rhoVAS
  Mux : Mux  Inputs=2
  Sum2 : Sum  Inputs=|+-
  Sum3 : Sum  Inputs=-+|
  Sum4 : Sum  Inputs=+-
  Sum5 : Sum  Inputs=|++
  length change term : Trigonometry
  offset correction term : Trigonometry
  variable lever term : Trigonometry  Operator=cos
  lmtu [m] : Outport  VectorParamsAs1DForOutWhenUnconnected=on
  lever [m] : Outport  Port=2  VectorParamsAs1DForOutWhenUnconnected=on
  wires:
  phi23 [rad]/1 -> Sum3/2
  Sum3/1 -> variable lever term/1, length change term/1
  Constant3/1 -> Sum3/1, Sum2/2
  Sum2/1 -> offset correction term/1
  Constant2/1 -> Sum2/1
  length change term/1 -> Sum4/2
  offset correction term/1 -> Sum4/1
  Sum4/1 -> Mux/1
  Constant/1 -> Sum5/1
  Sum5/1 -> lmtu [m]/1
  Gain4/1 -> Sum5/2
  variable lever term/1 -> Mux/2
  Mux/1 -> Gain2/1
  Gain2/1 -> Demux/1
  Demux/1 -> Gain4/1
  Demux/2 -> lever [m]/1

== system nms_model_Push/Muscle Actuation Layer/R Ankle Joint Limits ==
  note: Ankle Joint Limits
  phi [rad] : Inport
  dphi [rad/s] : Inport  Port=2
  Gain1 : Gain  Gain=c_jointstop
  Gain2 : Gain  Gain=-1
  Gain3 : Gain  Gain=c_jointstop
  Gain4 : Gain  Gain=1/w_max_jointstop
  Limit Ankle Range : simulink/Logic and Bit Operations/Interval Test  IntervalClosedRight=on  uplimit=phi12_UpLimit + 40*pi/180  IntervalClosedLeft=on  lowlimit=phi12_LowLimit - 40*pi/180  OutDataTypeStr=boolean
  Logical Operator3 : Logic  Operator=NOT  AllPortsSameDT=off  OutDataTypeStr=boolean
  Mux1 : Mux  Inputs=2
  Mux3 : Mux  Inputs=2
  Overextension Torque : Fcn  Expr="- u(1)  *  (1-u(2)) * (u(2)<1) * (u(1)>0)"
  Overflexion Torque : Fcn  Expr="- u(1)  *  (1-u(2)) * (u(2)<1) * (u(1)<0)"
  Stop Simulation1 : Stop
  Sum : Sum  Inputs=|+-
  Sum1 : Sum  Inputs=|+-
  Sum2 : Sum
  overextension angle : Constant  Value=phi12_UpLimit
  overflexion angle : Constant  Value=phi12_LowLimit
  M_stop [Nm] : Outport  VectorParamsAs1DForOutWhenUnconnected=on
  wires:
  Mux3/1 -> Overextension Torque/1
  Gain3/1 -> Mux3/1
  dphi [rad/s]/1 -> Gain4/1
  overextension angle/1 -> Sum/2
  phi [rad]/1 -> Sum/1, Sum1/1, Limit Ankle Range/1
  Sum/1 -> Gain3/1
  Gain4/1 -> Gain2/1, Mux1/2
  Gain1/1 -> Mux1/1
  Sum1/1 -> Gain1/1
  overflexion angle/1 -> Sum1/2
  Mux1/1 -> Overflexion Torque/1
  Sum2/1 -> M_stop [Nm]/1
  Gain2/1 -> Mux3/2
  Overflexion Torque/1 -> Sum2/2
  Overextension Torque/1 -> Sum2/1
  Limit Ankle Range/1 -> Logical Operator3/1
  Logical Operator3/1 -> Stop Simulation1/1

== system nms_model_Push/Muscle Actuation Layer/R GAS ==
  note: SOLEUS Muscle-Tendon Dynamics
  note: Excitation Contraction Coupling
  STIM : Inport
  lmtc [m] : Inport  Port=2
  1 : Product  Inputs=**  SaturateOnIntegerOverflow=on  InputSameDT=on  OutDataTypeStr=Inherit: Same as first input
  1/lslack : Gain  Gain=1/lslackGAS  SaturateOnIntegerOverflow=on  OutDataTypeStr=Inherit: Same as input  ParamDataTypeStr=Inherit: Same as input
  BE force-length relation : Subsystem
  CE force-length relation : Subsystem
  CE inverse force-velocity relation : Subsystem
  Constant : Constant  Value=lslackGAS
  ECC TransferFcn : simulink_extras/Additional Linear/Transfer Fcn (with initial outputs)  N=[1]  D="[tau  1]"  Y0=preA  U0=0
      settings: AttributesFormatString=pre-activation: %<Y0>
  Fmax : Gain  Gain=FmaxGAS  SaturateOnIntegerOverflow=on  OutDataTypeStr=Inherit: Same as input  ParamDataTypeStr=Inherit: Same as input
  Fv = Fse / (A*Fce) : Product  Inputs=*/  SaturateOnIntegerOverflow=on  InputSameDT=on  OutDataTypeStr=Inherit: Same as first input
  Integrator : Integrator  InitialConditionSource=external  LowerSaturationLimit=0.05
  PE force-length relation : Subsystem
  SE force-length relation : Subsystem
  Sum : Sum  Inputs=|+-  SaturateOnIntegerOverflow=on  InputSameDT=on  OutDataTypeStr=Inherit: Same as first input
  Sum2 : Sum  Inputs=|-+  SaturateOnIntegerOverflow=on  InputSameDT=on  OutDataTypeStr=Inherit: Same as first input
  Sum3 : Sum  SaturateOnIntegerOverflow=on  InputSameDT=on  OutDataTypeStr=Inherit: Same as first input
  Sum4 : Sum  SaturateOnIntegerOverflow=on  InputSameDT=on  OutDataTypeStr=Inherit: Same as first input
  lce/lopt : Gain  Gain=1/loptGAS  SaturateOnIntegerOverflow=on  OutDataTypeStr=Inherit: Same as input  ParamDataTypeStr=Inherit: Same as input
  vmax*lopt : Gain  Gain=vmaxGAS*loptGAS  SaturateOnIntegerOverflow=on  OutDataTypeStr=Inherit: Same as input  ParamDataTypeStr=Inherit: Same as input
  Fmtc : Outport  InitialOutput=0  VectorParamsAs1DForOutWhenUnconnected=on
  Lce : Outport  Port=2  InitialOutput=0  VectorParamsAs1DForOutWhenUnconnected=on
  Vce : Outport  Port=3  InitialOutput=0  VectorParamsAs1DForOutWhenUnconnected=on
  Lse : Outport  Port=4  InitialOutput=0  VectorParamsAs1DForOutWhenUnconnected=on
  A : Outport  Port=5  InitialOutput=0  VectorParamsAs1DForOutWhenUnconnected=on
  wires:
  Integrator/1 -> Sum/2, lce/lopt/1, Lce/1  "lce"
  Sum/1 -> 1/lslack/1, Lse/1  "lse"
  lce/lopt/1 -> CE force-length relation/1(lce [lopt]), BE force-length relation/1(lce [lopt]), PE force-length relation/1(lce [lopt])
  Fv = Fse / (A*Fce)/1 -> CE inverse force-velocity relation/1(Fv[Fmax])  "fv"
  vmax*lopt/1 -> Integrator/1, Vce/1  "vce"
  lmtc [m]/1 -> Sum2/2, Sum/1  "lmtc"
  Fmax/1 -> Fmtc/1  "Fmtc"
  1/lslack/1 -> SE force-length relation/1(lse [lslack])
  SE force-length relation/1(fse [Fmax]) -> Fmax/1, Sum4/1
  Sum2/1 -> Integrator/2
  Constant/1 -> Sum2/1
  CE force-length relation/1(fce [Fmax]) -> 1/1
  STIM/1 -> ECC TransferFcn/1
  Sum4/1 -> Fv = Fse / (A*Fce)/1
  PE force-length relation/1(fpe [Fmax]) -> Sum3/1
  1/1 -> Sum3/2
  BE force-length relation/1(fbe [Fmax]) -> Sum4/2
  Sum3/1 -> Fv = Fse / (A*Fce)/2
  CE inverse force-velocity relation/1(v[vmax]) -> vmax*lopt/1
  ECC TransferFcn/1 -> 1/2, A/1

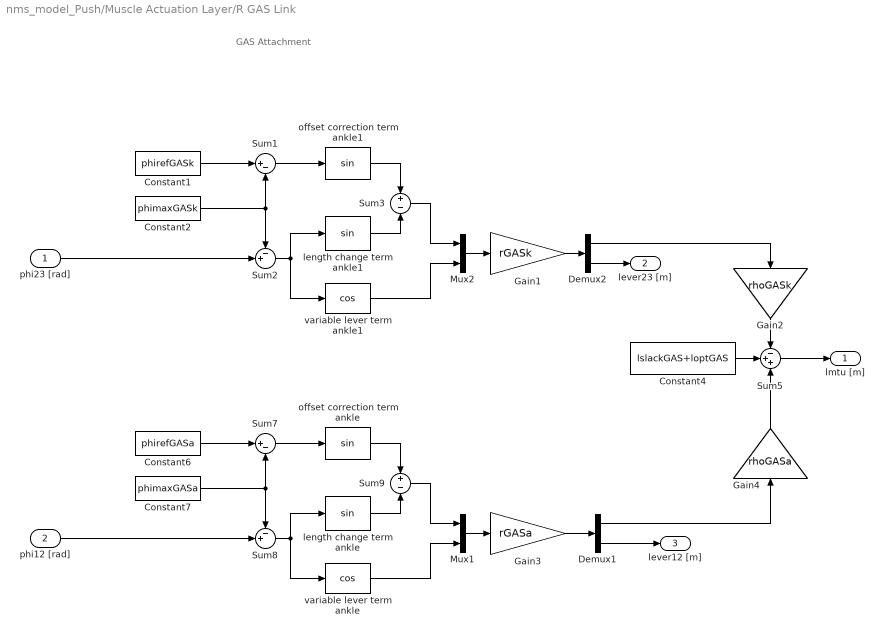
== system nms_model_Push/Muscle Actuation Layer/R GAS Link ==
  note: GAS Attachment
  phi23 [rad] : Inport
  phi12 [rad] : Inport  Port=2
  Constant1 : Constant  Value=phirefGASk
  Constant2 : Constant  Value=phimaxGASk
  Constant4 : Constant  Value=lslackGAS+loptGAS
  Constant6 : Constant  Value=phirefGASa
  Constant7 : Constant  Value=phimaxGASa
  Demux1 : Demux  Outputs=2
  Demux2 : Demux  Outputs=2
  Gain1 : Gain  Gain=rGASk
  Gain2 : Gain  Gain=rhoGASk
  Gain3 : Gain  Gain=rGASa
  Gain4 : Gain  Gain=rhoGASa
  Mux1 : Mux  Inputs=2
  Mux2 : Mux  Inputs=2
  Sum1 : Sum  Inputs=|+-
  Sum2 : Sum  Inputs=-+|
  Sum3 : Sum  Inputs=+-
  Sum5 : Sum  Inputs=-++
  Sum7 : Sum  Inputs=|+-
  Sum8 : Sum  Inputs=-+|
  Sum9 : Sum  Inputs=+-
  length change term ankle : Trigonometry
  length change term ankle1 : Trigonometry
  offset correction term ankle : Trigonometry
  offset correction term ankle1 : Trigonometry
  variable lever term ankle : Trigonometry  Operator=cos
  variable lever term ankle1 : Trigonometry  Operator=cos
  lmtu [m] : Outport  VectorParamsAs1DForOutWhenUnconnected=on
  lever23 [m] : Outport  Port=2  VectorParamsAs1DForOutWhenUnconnected=on
  lever12 [m] : Outport  Port=3  VectorParamsAs1DForOutWhenUnconnected=on
  wires:
  phi12 [rad]/1 -> Sum8/2
  Sum5/1 -> lmtu [m]/1
  variable lever term ankle/1 -> Mux1/2
  Demux1/2 -> lever12 [m]/1
  Sum8/1 -> variable lever term ankle/1, length change term ankle/1
  Constant7/1 -> Sum8/1, Sum7/2
  Sum7/1 -> offset correction term ankle/1
  Constant6/1 -> Sum7/1
  length change term ankle/1 -> Sum9/2
  offset correction term ankle/1 -> Sum9/1
  Sum9/1 -> Mux1/1
  Constant4/1 -> Sum5/2
  Mux1/1 -> Gain3/1
  Gain3/1 -> Demux1/1
  Demux1/1 -> Gain4/1
  Gain4/1 -> Sum5/3
  phi23 [rad]/1 -> Sum2/2
  variable lever term ankle1/1 -> Mux2/2
  Sum2/1 -> variable lever term ankle1/1, length change term ankle1/1
  Constant2/1 -> Sum2/1, Sum1/2
  Sum1/1 -> offset correction term ankle1/1
  Constant1/1 -> Sum1/1
  length change term ankle1/1 -> Sum3/2
  offset correction term ankle1/1 -> Sum3/1
  Sum3/1 -> Mux2/1
  Mux2/1 -> Gain1/1
  Gain1/1 -> Demux2/1
  Demux2/2 -> lever23 [m]/1
  Demux2/1 -> Gain2/1
  Gain2/1 -> Sum5/1

== system nms_model_Push/Muscle Actuation Layer/R GLU ==
  note: SOLEUS Muscle-Tendon Dynamics
  note: Excitation Contraction Coupling
  STIM : Inport
  lmtc [m] : Inport  Port=2
  1 : Product  Inputs=**  SaturateOnIntegerOverflow=on  InputSameDT=on  OutDataTypeStr=Inherit: Same as first input
  1/lslack : Gain  Gain=1/lslackGLU  SaturateOnIntegerOverflow=on  OutDataTypeStr=Inherit: Same as input  ParamDataTypeStr=Inherit: Same as input
  BE force-length relation : Subsystem
  CE force-length relation : Subsystem
  CE inverse force-velocity relation : Subsystem
  Constant : Constant  Value=lslackGLU
  ECC TransferFcn : simulink_extras/Additional Linear/Transfer Fcn (with initial outputs)  N=[1]  D="[tau  1]"  Y0=preA  U0=0
      settings: AttributesFormatString=pre-activation: %<Y0>
  Fmax : Gain  Gain=FmaxGLU  SaturateOnIntegerOverflow=on  OutDataTypeStr=Inherit: Same as input  ParamDataTypeStr=Inherit: Same as input
  Fv = Fse / (A*Fce) : Product  Inputs=*/  SaturateOnIntegerOverflow=on  InputSameDT=on  OutDataTypeStr=Inherit: Same as first input
  Integrator : Integrator  InitialConditionSource=external  LowerSaturationLimit=0.05
  PE force-length relation : Subsystem
  SE force-length relation : Subsystem
  Sum : Sum  Inputs=|+-  SaturateOnIntegerOverflow=on  InputSameDT=on  OutDataTypeStr=Inherit: Same as first input
  Sum2 : Sum  Inputs=|-+  SaturateOnIntegerOverflow=on  InputSameDT=on  OutDataTypeStr=Inherit: Same as first input
  Sum3 : Sum  SaturateOnIntegerOverflow=on  InputSameDT=on  OutDataTypeStr=Inherit: Same as first input
  Sum4 : Sum  SaturateOnIntegerOverflow=on  InputSameDT=on  OutDataTypeStr=Inherit: Same as first input
  lce/lopt : Gain  Gain=1/loptGLU  SaturateOnIntegerOverflow=on  OutDataTypeStr=Inherit: Same as input  ParamDataTypeStr=Inherit: Same as input
  vmax*lopt : Gain  Gain=vmaxGLU*loptGLU  SaturateOnIntegerOverflow=on  OutDataTypeStr=Inherit: Same as input  ParamDataTypeStr=Inherit: Same as input
  Fmtc : Outport  InitialOutput=0  VectorParamsAs1DForOutWhenUnconnected=on
  Lce : Outport  Port=2  InitialOutput=0  VectorParamsAs1DForOutWhenUnconnected=on
  Vce : Outport  Port=3  InitialOutput=0  VectorParamsAs1DForOutWhenUnconnected=on
  Lse : Outport  Port=4  InitialOutput=0  VectorParamsAs1DForOutWhenUnconnected=on
  A : Outport  Port=5  InitialOutput=0  VectorParamsAs1DForOutWhenUnconnected=on
  wires:
  Integrator/1 -> Sum/2, lce/lopt/1, Lce/1  "lce"
  Sum/1 -> 1/lslack/1, Lse/1  "lse"
  lce/lopt/1 -> CE force-length relation/1(lce [lopt]), BE force-length relation/1(lce [lopt]), PE force-length relation/1(lce [lopt])
  Fv = Fse / (A*Fce)/1 -> CE inverse force-velocity relation/1(Fv[Fmax])  "fv"
  vmax*lopt/1 -> Integrator/1, Vce/1  "vce"
  lmtc [m]/1 -> Sum2/2, Sum/1  "lmtc"
  Fmax/1 -> Fmtc/1  "Fmtc"
  1/lslack/1 -> SE force-length relation/1(lse [lslack])
  SE force-length relation/1(fse [Fmax]) -> Fmax/1, Sum4/1
  Sum2/1 -> Integrator/2
  Constant/1 -> Sum2/1
  CE force-length relation/1(fce [Fmax]) -> 1/1
  Sum4/1 -> Fv = Fse / (A*Fce)/1
  PE force-length relation/1(fpe [Fmax]) -> Sum3/1
  1/1 -> Sum3/2
  BE force-length relation/1(fbe [Fmax]) -> Sum4/2
  Sum3/1 -> Fv = Fse / (A*Fce)/2
  CE inverse force-velocity relation/1(v[vmax]) -> vmax*lopt/1
  STIM/1 -> ECC TransferFcn/1
  ECC TransferFcn/1 -> 1/2, A/1

== system nms_model_Push/Muscle Actuation Layer/R GLU Link ==
  note: GLUTEUS Attachment
  phi34 [rad] : Inport
  Constant : Constant  Value=lslackGLU+loptGLU
  Constant1 : Constant  Value=rGLU
  Constant2 : Constant  Value=phirefGLU
  Gain2 : Gain  Gain=rhoGLU
  Product : Product  RndMeth=Zero
  Sum2 : Sum  Inputs=|+-
  Sum5 : Sum  Inputs=|+-
  lmtu [m] : Outport  VectorParamsAs1DForOutWhenUnconnected=on
  lever [m] : Outport  Port=2  VectorParamsAs1DForOutWhenUnconnected=on
  wires:
  Constant/1 -> Sum5/1
  Sum5/1 -> lmtu [m]/1
  Product/1 -> Gain2/1
  phi34 [rad]/1 -> Sum2/1
  Constant2/1 -> Sum2/2
  Sum2/1 -> Product/1
  Constant1/1 -> Product/2, lever [m]/1
  Gain2/1 -> Sum5/2
